simulink model "XeCanBangLR"  (R2022b)
settings: Solver=FixedStepAuto  StartTime=0.0  StopTime=50  FixedStep=0.01  RelTol=1e-3
settings Model: Creator=Admins  LastModifiedBy=Admins
settings DataIOCC: ReturnWorkspaceOutputs=off

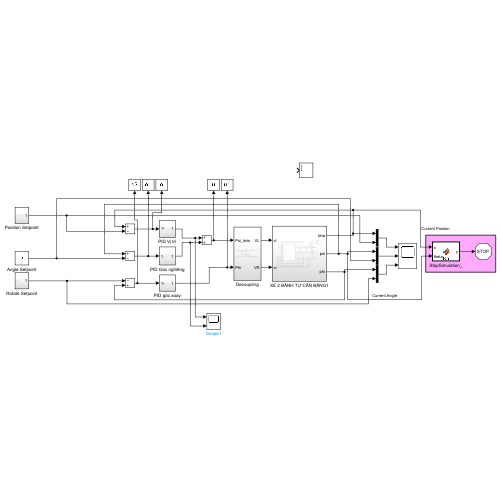
[thumbnail: Simulink's stored preview of the top-level diagram]
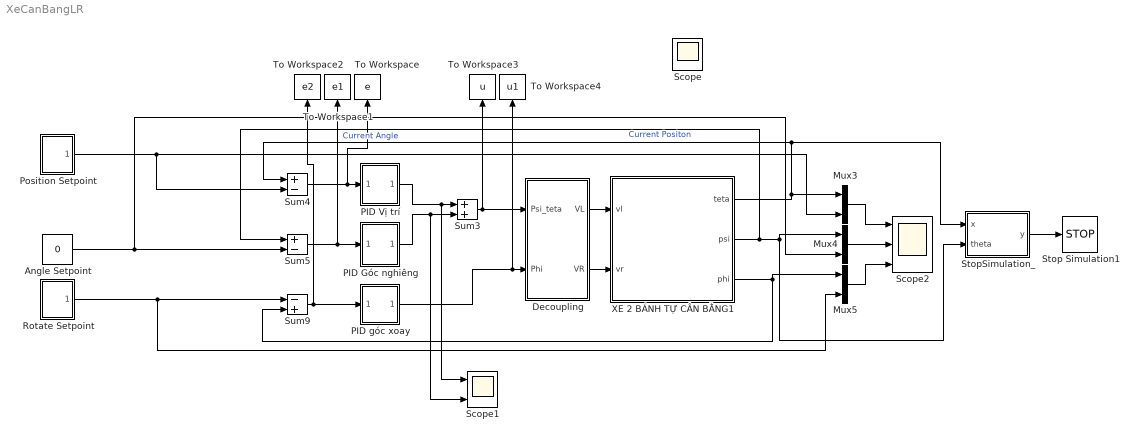
== system XeCanBangLR ==
  Angle Setpoint : Constant  Value=0
  Decoupling : Subsystem
  Mux3 : Mux  Inputs=2
  Mux4 : Mux  Inputs=2
  Mux5 : Mux  Inputs=2
  PID Góc nghiêng : Subsystem
  PID Vị trí : Subsystem
  PID góc xoay : Subsystem
  Position Setpoint : Subsystem
  Rotate Setpoint : Subsystem
  Scope : Scope
  Scope1 : Scope  NumInputPorts=2
  Scope2 : Scope  NumInputPorts=3
  Stop Simulation1 : Stop
  StopSimulation_ : MATLAB Function  TreatAsAtomicUnit=on
  Sum3 : Sum
  Sum4 : Sum  Inputs=+|-
  Sum5 : Sum  Inputs=+-
  Sum9 : Sum  Inputs=-+
  To Workspace : ToWorkspace  VariableName=e  SampleTime=-1
  To Workspace1 : ToWorkspace  VariableName=e1  SampleTime=-1
  To Workspace2 : ToWorkspace  VariableName=e2  SampleTime=-1
  To Workspace3 : ToWorkspace  VariableName=u  SampleTime=-1
  To Workspace4 : ToWorkspace  VariableName=u1  SampleTime=-1
  XE 2 BÁNH TỰ CÂN BẰNG1 : Subsystem
  wires:
  PID Góc nghiêng/1(Out1) -> Scope1/2, Sum3/2
  Position Setpoint/1(Out1) -> Mux3/2, Sum4/2
  Angle Setpoint/1 -> Sum5/2, Mux4/2
  XE 2 BÁNH TỰ CÂN BẰNG1/3(phi) -> Mux5/1, Sum9/2
  PID Vị trí/1(Out1) -> Scope1/1, Sum3/1
  Sum4/1 -> To Workspace/1, PID Vị trí/1(In1)
  Rotate Setpoint/1(Out1) -> Mux5/2, Sum9/1
  Mux4/1 -> Scope2/2
  Mux5/1 -> Scope2/3
  Sum5/1 -> PID Góc nghiêng/1(In1), To Workspace1/1
  Sum3/1 -> Decoupling/1(Psi_teta), To Workspace3/1
  Sum9/1 -> PID góc xoay/1(In1), To Workspace2/1
  Mux3/1 -> Scope2/1
  XE 2 BÁNH TỰ CÂN BẰNG1/1(teta) -> StopSimulation_/1(x), Sum4/1, Mux3/1  "Current Positon"
  XE 2 BÁNH TỰ CÂN BẰNG1/2(psi) -> Sum5/1, Mux4/1, StopSimulation_/2(theta)  "Current Angle"
  StopSimulation_/1(y) -> Stop Simulation1/1
  PID góc xoay/1(Out1) -> To Workspace4/1, Decoupling/2(Phi)
  Decoupling/1(VL) -> XE 2 BÁNH TỰ CÂN BẰNG1/1(vl)
  Decoupling/2(VR) -> XE 2 BÁNH TỰ CÂN BẰNG1/2(vr)

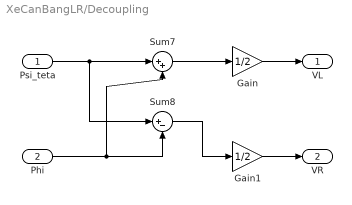
== system XeCanBangLR/Decoupling ==
  Psi_teta : Inport
  Phi : Inport  Port=2
  Gain : Gain  Gain=1/2
  Gain1 : Gain  Gain=1/2
  Sum7 : Sum  Inputs=|++
  Sum8 : Sum  Inputs=|+-
  VL : Outport
  VR : Outport  Port=2
  wires:
  Phi/1 -> Sum8/2, Sum7/2
  Psi_teta/1 -> Sum8/1, Sum7/1
  Sum7/1 -> Gain/1
  Sum8/1 -> Gain1/1
  Gain/1 -> VL/1
  Gain1/1 -> VR/1

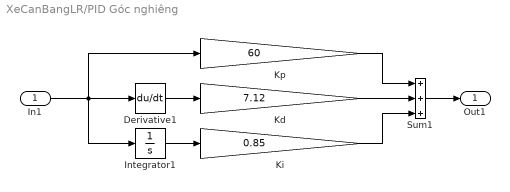
== system XeCanBangLR/PID Góc nghiêng ==
  In1 : Inport
  Derivative1 : Derivative
  Integrator1 : Integrator
  Kd : Gain  Gain=7.12
  Ki : Gain  Gain=0.85
  Kp : Gain  Gain=60
  Sum1 : Sum  Inputs=+++
  Out1 : Outport
  wires:
  Ki/1 -> Sum1/3
  In1/1 -> Kp/1, Integrator1/1, Derivative1/1
  Integrator1/1 -> Ki/1
  Derivative1/1 -> Kd/1
  Kp/1 -> Sum1/1
  Kd/1 -> Sum1/2
  Sum1/1 -> Out1/1

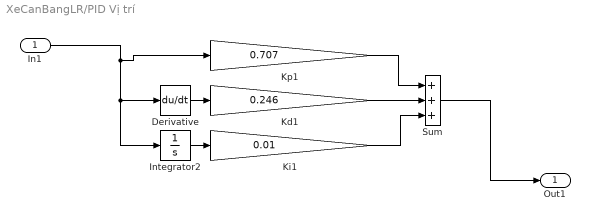
== system XeCanBangLR/PID Vị trí ==
  In1 : Inport
  Derivative : Derivative
  Integrator2 : Integrator
  Kd1 : Gain  Gain=0.246
  Ki1 : Gain  Gain=0.01
  Kp1 : Gain  Gain=0.707
  Sum : Sum  Inputs=+++
  Out1 : Outport
  wires:
  In1/1 -> Integrator2/1, Derivative/1, Kp1/1
  Sum/1 -> Out1/1
  Derivative/1 -> Kd1/1
  Kp1/1 -> Sum/1
  Integrator2/1 -> Ki1/1
  Kd1/1 -> Sum/2
  Ki1/1 -> Sum/3

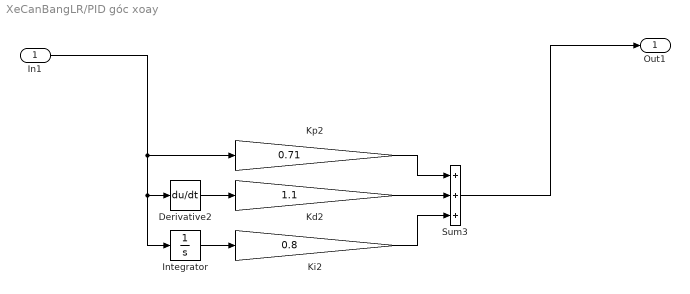
== system XeCanBangLR/PID góc xoay ==
  In1 : Inport
  Derivative2 : Derivative
  Integrator : Integrator
  Kd2 : Gain  Gain=1.1
  Ki2 : Gain  Gain=0.8
  Kp2 : Gain  Gain=0.71
  Sum3 : Sum  Inputs=+++
  Out1 : Outport
  wires:
  Derivative2/1 -> Kd2/1
  In1/1 -> Integrator/1, Derivative2/1, Kp2/1
  Kd2/1 -> Sum3/2
  Ki2/1 -> Sum3/3
  Integrator/1 -> Ki2/1
  Sum3/1 -> Out1/1
  Kp2/1 -> Sum3/1

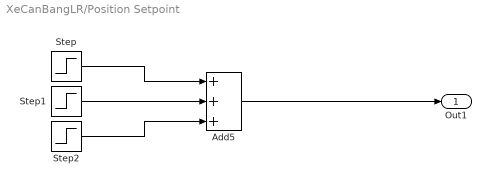
== system XeCanBangLR/Position Setpoint ==
  Add5 : Sum  Inputs=+++
  Step : Step  Time=0  SampleTime=0
  Step1 : Step  Time=20  After=-1.5  SampleTime=0
  Step2 : Step  Time=35  After=3  SampleTime=0
  Out1 : Outport
  wires:
  Step1/1 -> Add5/2
  Step/1 -> Add5/1
  Step2/1 -> Add5/3
  Add5/1 -> Out1/1

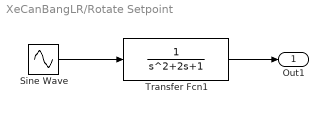
== system XeCanBangLR/Rotate Setpoint ==
  Sine Wave : Sin  Amplitude=0.06  Frequency=pi/12  SampleTime=0
  Transfer Fcn1 : TransferFcn
  Out1 : Outport
  wires:
  Transfer Fcn1/1 -> Out1/1
  Sine Wave/1 -> Transfer Fcn1/1

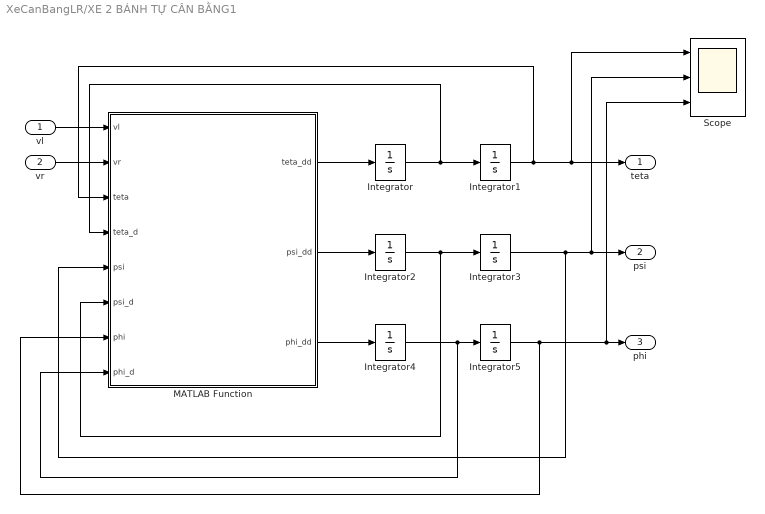
== system XeCanBangLR/XE 2 BÁNH TỰ CÂN BẰNG1 ==
  vl : Inport
  vr : Inport  Port=2
  Integrator{,1..5} (6 alike) : Integrator
  MATLAB Function : MATLAB Function  TreatAsAtomicUnit=on
  Scope : Scope  NumInputPorts=3
  teta : Outport
  psi : Outport  Port=2
  phi : Outport  Port=3
  wires:
  Integrator/1 -> MATLAB Function/4(teta_d), Integrator1/1
  Integrator1/1 -> MATLAB Function/3(teta), Scope/1, teta/1
  MATLAB Function/1(teta_dd) -> Integrator/1
  Integrator3/1 -> MATLAB Function/5(psi), Scope/2, psi/1
  Integrator2/1 -> MATLAB Function/6(psi_d), Integrator3/1
  MATLAB Function/2(psi_dd) -> Integrator2/1
  Integrator5/1 -> MATLAB Function/7(phi), Scope/3, phi/1
  Integrator4/1 -> MATLAB Function/8(phi_d), Integrator5/1
  MATLAB Function/3(phi_dd) -> Integrator4/1
  vl/1 -> MATLAB Function/1(vl)
  vr/1 -> MATLAB Function/2(vr)

== matlab function XeCanBangLR/XE 2 BÁNH TỰ CÂN BẰNG1/MATLAB Function ==
  data: vl input; teta_dd output; vr input; teta input; teta_d input; psi input; psi_d input; phi input; phi_d input; psi_dd output; phi_dd output
function [teta_dd,psi_dd,phi_dd] = fcn(vl  ,vr  ,teta,teta_d,psi,psi_d,phi,phi_d)

%% Thông số hệ thống xe 2 bánh tự cân bằng dùng LQR
m = 0.08; %Khoi luong banh xe
M = 0.7; %Khoi luong robot
R = 0.0325; %ban kinh ban xe
W = 0.15; %Chieu rong robot
D = 0.06; %Chieu sau robot
H = 0.13; %Chieu cao robot
L = 0.02; %khoang cach tu trong tam den truc banh xe
fw = 0.001; %He so ma sat giua banh xe voi mat phang
fm = 0.001; %he so ma sat giua dong co va robot
Jm = 0.00045; %moment quan tinh cua dong co
Jw = m*R^2/2;
J_psi = M*L^2/3;
J_phi = M*(W^2+D^2)/12;
Rm = 14.6; %Dien tro dong co DC
Kb = 0.0218; %he so emf cua dong co
Kt = 0.8; %Momen xoan cua dong co DC
n = 30; %Ty so giam toc
g = 9.81; %Gia toc trong truong
alpha = n*Kt/Rm; beta=n*Kt*Kb/Rm+fm; a =alpha;
T=0.01;

teta_dd = (J_psi*a*vl*2 + J_psi*a*vr*2 - 2*J_psi*beta*teta_d + 2*J_psi*beta*psi_d - 2*J_psi*fw*teta_d + L^2*M*a*vl*2 + L^2*M*a*vr*2 - 2*L^2*M*beta*teta_d + 2*L^2*M*beta*psi_d - 2*L^2*M*fw*teta_d - 4*Jm*fw*n^2*teta_d + L^3*M^2*R*psi_d^2*sin(psi) - 2*L*M*R*beta*teta_d*cos(psi) + 2*L*M*R*beta*psi_d*cos(psi) - L^3*M^2*R*phi_d^2*cos(psi)^2*sin(psi) - L^2*M^2*R*g*cos(psi)*sin(psi) + J_psi*L*M*R*psi_d^2*sin(psi) + 2*Jm*L*M*g*n^2*sin(psi) + L*M*R*a*vl*2*cos(psi) + L*M*R*a*vr*2*cos(psi) + 2*Jm*L^2*M*n^2*phi_d^2*cos(psi)*sin(psi) + 2*Jm*L*M*R*n^2*psi_d^2*sin(psi))/(2*J_psi*Jw + L^2*M^2*R^2 + 2*Jw*L^2*M + J_psi*M*R^2 + 2*J_psi*Jm*n^2 + 4*Jm*Jw*n^2 + 2*J_psi*R^2*m + 2*Jm*L^2*M*n^2 + 2*Jm*M*R^2*n^2 + 2*L^2*M*R^2*m + 4*Jm*R^2*m*n^2 - L^2*M^2*R^2*cos(psi)^2 + 4*Jm*L*M*R*n^2*cos(psi));
psi_dd = -(2*Jw*a*vl*2 + 2*Jw*a*vr*2 - 4*Jw*beta*teta_d + 4*Jw*beta*psi_d + M*R^2*a*vl*2 + M*R^2*a*vr*2 - 2*M*R^2*beta*teta_d + 2*M*R^2*beta*psi_d + 2*R^2*a*m*vl*2 + 2*R^2*a*m*vr*2 + 4*Jm*fw*n^2*teta_d - 4*R^2*beta*m*teta_d + 4*R^2*beta*m*psi_d - L*M^2*R^2*g*sin(psi) - 2*Jw*L*M*g*sin(psi) - 2*L*M*R*beta*teta_d*cos(psi) + 2*L*M*R*beta*psi_d*cos(psi) - 2*L*M*R*fw*teta_d*cos(psi) + L^2*M^2*R^2*psi_d^2*cos(psi)*sin(psi) - L^2*M^2*R^2*phi_d^2*cos(psi)*sin(psi) - 2*Jw*L^2*M*phi_d^2*cos(psi)*sin(psi) - 2*Jm*L*M*g*n^2*sin(psi) - 2*L*M*R^2*g*m*sin(psi) + L*M*R*a*vl*2*cos(psi) + L*M*R*a*vr*2*cos(psi) - 2*Jm*L^2*M*n^2*phi_d^2*cos(psi)*sin(psi) - 2*L^2*M*R^2*m*phi_d^2*cos(psi)*sin(psi) - 2*Jm*L*M*R*n^2*psi_d^2*sin(psi))/(2*J_psi*Jw + L^2*M^2*R^2 + 2*Jw*L^2*M + J_psi*M*R^2 + 2*J_psi*Jm*n^2 + 4*Jm*Jw*n^2 + 2*J_psi*R^2*m + 2*Jm*L^2*M*n^2 + 2*Jm*M*R^2*n^2 + 2*L^2*M*R^2*m + 4*Jm*R^2*m*n^2 - L^2*M^2*R^2*cos(psi)^2 + 4*Jm*L*M*R*n^2*cos(psi));
phi_dd = -(W^2*beta*phi_d + W^2*fw*phi_d + R*W*a*vl*2 - R*W*a*vr*2 + 4*L^2*M*R^2*psi_d*phi_d*cos(psi)*sin(psi))/(2*J_phi*R^2 + Jm*W^2 + Jm*W^2*n^2 + R^2*W^2*m + 2*L^2*M*R^2*sin(psi)^2);

== matlab function XeCanBangLR/StopSimulation_ ==
  data: x input; y output; theta input
function y = fcn(x,theta)
if (abs(x)> 3)||(abs(theta)*180/pi > 15)
    y=1;
else
    y=0;
end
